simulink model "SImulink_Modell_Aufgabe_22"  (R2017b)
settings: Solver=VariableStepAuto  StartTime=0.0  StopTime=10.0  RelTol=1e-3
values from neighbouring files (symbols this model uses):
  A = double(vpa(A))    [Skript_Vorbereitung.m]
  Ar11 = Ar(1:n,1:n)    [Skript_Vorbereitung.m]
  Ar12 = Ar(1:n,n+1:length(A))    [Skript_Vorbereitung.m]
  Ar21 = Ar(n+1:length(A), 1:n)    [Skript_Vorbereitung.m]
  Ar22 = Ar(n+1:length(A),n+1:length(A))    [Skript_Vorbereitung.m]
  b = double(vpa(b))    [Skript_Vorbereitung.m]
  br1 = br(1:n)    [Skript_Vorbereitung.m]
  br2 = br(n+1:length(A))    [Skript_Vorbereitung.m]
  C = [1 0 0 0; 0 0 1 0]    [Skript_Vorbereitung.m]
  C_a = double([1 0 -1 0])    [Skript_Vorbereitung.m]
  k = acker(A,b,p)    [Skript_Vorbereitung.m]
  L_red = L_riccati_red    [Skript_Vorbereitung.m]
  L_voll = L_riccati    [Skript_Vorbereitung.m]
  vorFilter = -inv(C_a*inv(A-b*k)*b)    [Skript_Vorbereitung.m]
settings Model: Creator=Lucas  LastModifiedBy=Lucas

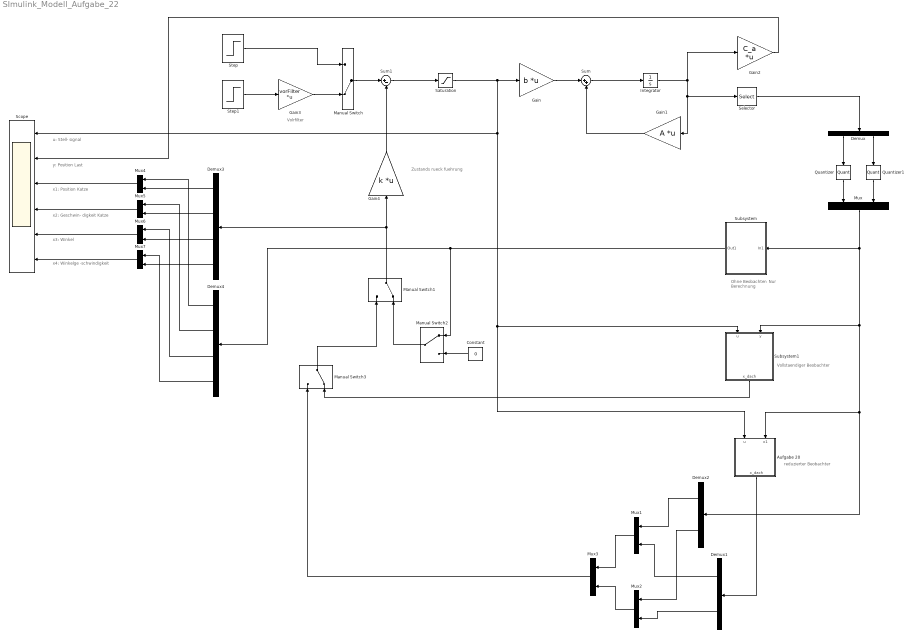
== system SImulink_Modell_Aufgabe_22 ==
  note: x4: Winkelge
      | -schwindigkeit
  note: x3: Winkel
  note: x2: Geschwin-
      | digkeit Katze
  note: x1: Position
      | Katze
  note: y: Position
      | Last
  note: u: Stell-
      | signal
  note: Zustands
      | rueck
      | fuehrung
  note: Volrfilter
  note: Ohne Beobachter:
      | Nur Berechnung
  note: Vollstaendiger
      | Beobachter
  note: reduzierter
      | Beobachter
  Aufgabe 20 : Subsystem
  Constant : Constant  Value=0
  Demux : Demux  Outputs=2
  Demux1 : Demux  Outputs=2
  Demux2 : Demux  Outputs=2
  Demux3 : Demux
  Demux4 : Demux
  Gain : Gain  Gain=b  Multiplication=Matrix(K*u)
  Gain1 : Gain  Gain=A  Multiplication=Matrix(K*u)
  Gain2 : Gain  Gain=C_a  Multiplication=Matrix(K*u)
  Gain3 : Gain  Gain=vorFilter  Multiplication=Matrix(K*u)
  Gain4 : Gain  Gain=k  Multiplication=Matrix(K*u)
  Integrator : Integrator
  Manual Switch : ManualSwitch  CurrentSetting=0
  Manual Switch1 : ManualSwitch  CurrentSetting=0
  Manual Switch2 : ManualSwitch
  Manual Switch3 : ManualSwitch  CurrentSetting=0
  Mux{,1..7} (8 alike) : Mux  Inputs=2
  Quantizer : Quantizer
  Quantizer1 : Quantizer
  Saturation : Saturate  UpperLimit=10  LowerLimit=-10
  Scope : Scope  NumInputPorts=6
  Selector : Selector  InputPortWidth=4  IndexOptions=Index vector (dialog)  Indices=[1 3]  OutputSizes=1
  Step : Step  SampleTime=0
  Step1 : Step  SampleTime=0
  Subsystem : Subsystem
  Subsystem1 : Subsystem
  Sum : Sum  Inputs=|++
  Sum1 : Sum  Inputs=|+-
  wires:
  Gain/1 -> Sum/1
  Sum/1 -> Integrator/1
  Gain1/1 -> Sum/2
  Integrator/1 -> Gain2/1, Selector/1, Gain1/1
  Demux/1 -> Quantizer/1
  Selector/1 -> Demux/1
  Demux/2 -> Quantizer1/1
  Quantizer/1 -> Mux/1
  Quantizer1/1 -> Mux/2
  Mux/1 -> Demux2/1, Aufgabe 20/2(x1), Subsystem1/2(y), Subsystem/1(In1)
  Saturation/1 -> Scope/1, Aufgabe 20/1(u), Subsystem1/1(u), Gain/1
  Aufgabe 20/1(x_dach) -> Demux1/1
  Demux2/1 -> Mux1/1
  Demux1/1 -> Mux1/2
  Demux2/2 -> Mux2/1
  Demux1/2 -> Mux2/2
  Mux1/1 -> Mux3/1
  Mux2/1 -> Mux3/2
  Sum1/1 -> Saturation/1
  Manual Switch/1 -> Sum1/1
  Step/1 -> Manual Switch/1
  Gain3/1 -> Manual Switch/2
  Step1/1 -> Gain3/1
  Gain4/1 -> Sum1/2
  Manual Switch1/1 -> Demux3/1, Gain4/1
  Manual Switch2/1 -> Manual Switch1/2
  Subsystem/1(Out1) -> Manual Switch2/1, Demux4/1
  Constant/1 -> Manual Switch2/2
  Manual Switch3/1 -> Manual Switch1/1
  Subsystem1/1(x_dach) -> Manual Switch3/2
  Mux3/1 -> Manual Switch3/1
  Gain2/1 -> Scope/2
  Mux4/1 -> Scope/3
  Mux6/1 -> Scope/5
  Mux7/1 -> Scope/6
  Mux5/1 -> Scope/4
  Demux3/1 -> Mux4/2
  Demux3/2 -> Mux5/2
  Demux3/3 -> Mux6/2
  Demux3/4 -> Mux7/2
  Demux4/1 -> Mux4/1
  Demux4/2 -> Mux5/1
  Demux4/3 -> Mux6/1
  Demux4/4 -> Mux7/1

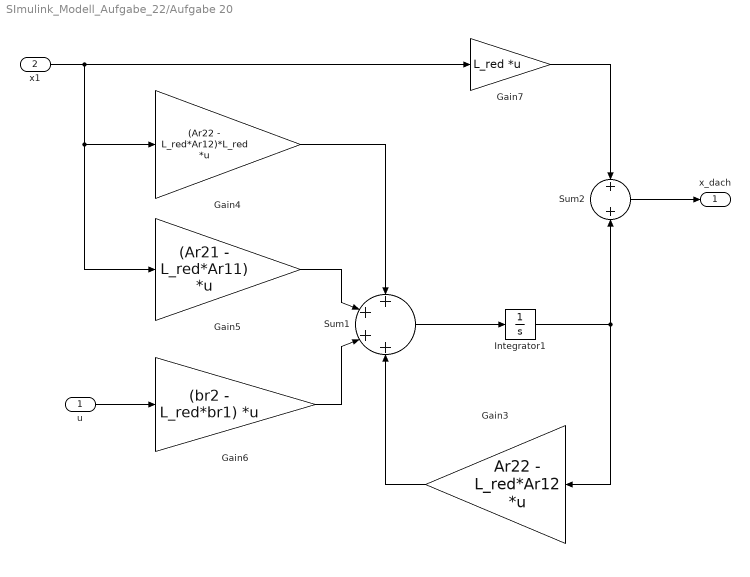
== system SImulink_Modell_Aufgabe_22/Aufgabe 20 ==
  u : Inport
  x1 : Inport  Port=2
  Gain3 : Gain  Gain=Ar22 - L_red*Ar12  Multiplication=Matrix(K*u)
  Gain4 : Gain  Gain=(Ar22 - L_red*Ar12)*L_red  Multiplication=Matrix(K*u)
  Gain5 : Gain  Gain=(Ar21 - L_red*Ar11)  Multiplication=Matrix(K*u)
  Gain6 : Gain  Gain=(br2 - L_red*br1)  Multiplication=Matrix(K*u)
  Gain7 : Gain  Gain=L_red  Multiplication=Matrix(K*u)
  Integrator1 : Integrator
  Sum1 : Sum  Inputs=++++
  Sum2 : Sum
  x_dach : Outport
  wires:
  Gain7/1 -> Sum2/1
  Sum1/1 -> Integrator1/1
  x1/1 -> Gain7/1, Gain5/1, Gain4/1
  Integrator1/1 -> Gain3/1, Sum2/2
  u/1 -> Gain6/1
  Gain3/1 -> Sum1/4
  Sum2/1 -> x_dach/1
  Gain5/1 -> Sum1/2
  Gain6/1 -> Sum1/3
  Gain4/1 -> Sum1/1

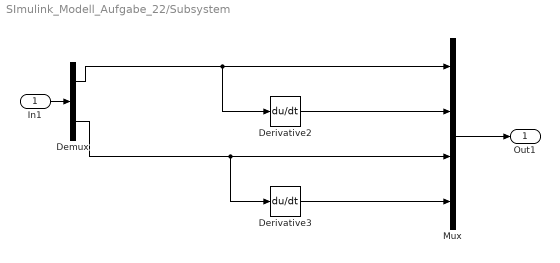
== system SImulink_Modell_Aufgabe_22/Subsystem ==
  In1 : Inport
  Demux : Demux  Outputs=2
  Derivative2 : Derivative
  Derivative3 : Derivative
  Mux : Mux
  Out1 : Outport
  wires:
  Demux/1 -> Mux/1, Derivative2/1
  Demux/2 -> Mux/3, Derivative3/1
  In1/1 -> Demux/1
  Mux/1 -> Out1/1
  Derivative2/1 -> Mux/2
  Derivative3/1 -> Mux/4

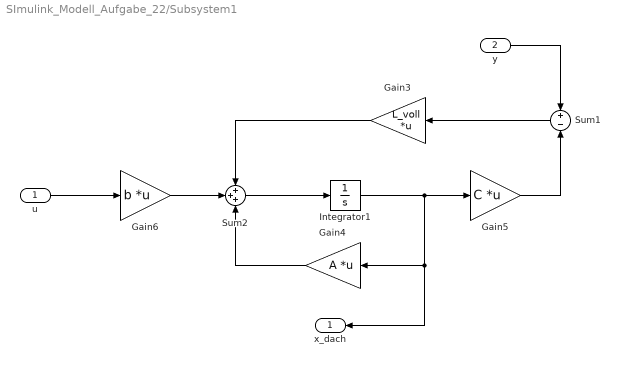
== system SImulink_Modell_Aufgabe_22/Subsystem1 ==
  u : Inport
  y : Inport  Port=2
  Gain3 : Gain  Gain=L_voll  Multiplication=Matrix(K*u)
  Gain4 : Gain  Gain=A  Multiplication=Matrix(K*u)
  Gain5 : Gain  Gain=C  Multiplication=Matrix(K*u)
  Gain6 : Gain  Gain=b  Multiplication=Matrix(K*u)
  Integrator1 : Integrator
  Sum1 : Sum  Inputs=+-
  Sum2 : Sum  Inputs=+++
  x_dach : Outport
  wires:
  Gain3/1 -> Sum2/1
  Sum2/1 -> Integrator1/1
  u/1 -> Gain6/1
  y/1 -> Sum1/1
  Integrator1/1 -> x_dach/1, Gain4/1, Gain5/1
  Gain5/1 -> Sum1/2
  Sum1/1 -> Gain3/1
  Gain4/1 -> Sum2/3
  Gain6/1 -> Sum2/2
